simulink library "nist_library"  (R2012b)
settings: Solver=VariableStepDiscrete  StartTime=0  StopTime=1000  RelTol=1e-3
undefined symbols (not defined in the file or in its folder): sfp, xlipgetpartsetting
libraries: xbsIndex_r4 x128, xps_library x10, nist_library x5, casper_library_misc x2, casper_library_delays x1
(part 1 of 3)
settings Model: RequirementInfo="{}  %GIDa_4c0522fd_96cd_4d16_968c_18936887b3dc"  Creator=root  LastModifiedBy=root

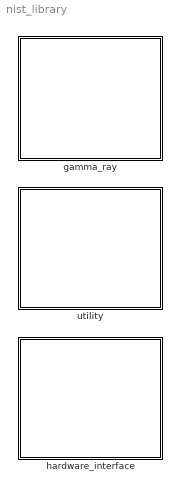
== system nist_library ==
  gamma_ray : Subsystem
  hardware_interface : Subsystem
  utility : Subsystem

== system nist_library/gamma_ray ==
  chan : Subsystem

== system nist_library/hardware_interface ==
  if_board : Subsystem
  tengbe : Subsystem

== system nist_library/utility ==
  complex_mult : Subsystem
  sync_extend : Subsystem
